simulink model "least_squares_parameter_id"  (R2022a)
settings: Solver=VariableStepAuto  StartTime=0.0  StopTime=10.0  RelTol=1e-3
libraries: simulink x1
settings Model: Creator=mluser  LastModifiedBy=mluser

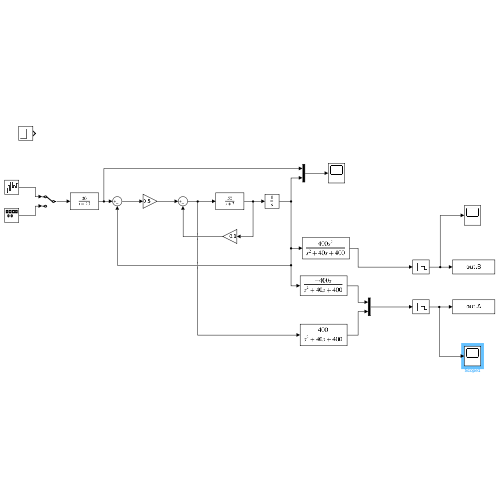
[thumbnail: Simulink's stored preview of the top-level diagram]
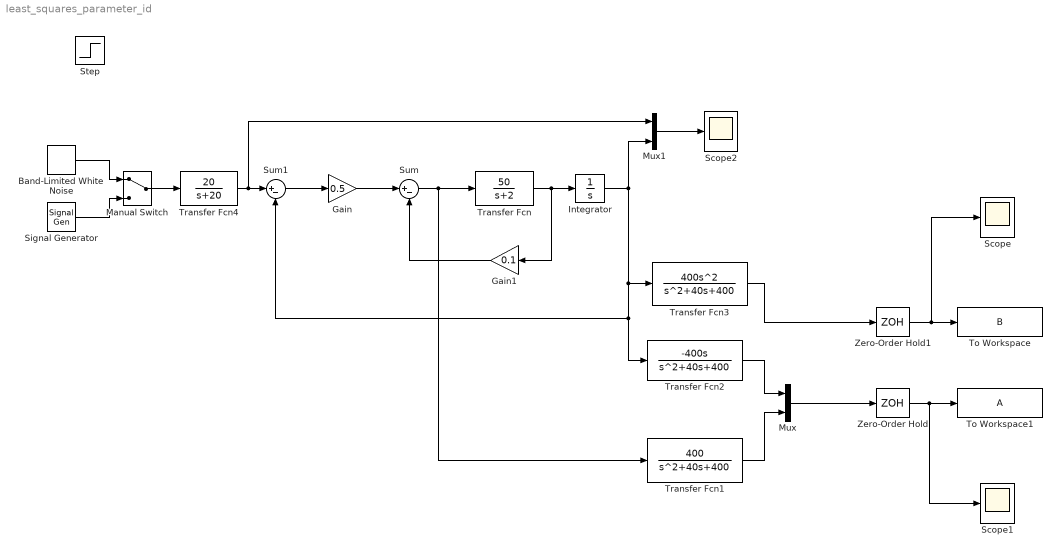
== system least_squares_parameter_id ==
  Band-Limited White Noise : simulink/Sources/Band-Limited White Noise  Cov=[0.1]  Ts=0.1  seed=[23341]
  Gain : Gain  Gain=0.5
  Gain1 : Gain  Gain=0.1
  Integrator : Integrator
  Manual Switch : ManualSwitch
  Mux : Mux  Inputs=2
  Mux1 : Mux  Inputs=2
  Scope : Scope
  Scope1 : Scope
  Scope2 : Scope
  Signal Generator : SignalGenerator  Units=rad/sec
  Step : Step  SampleTime=0
  Sum : Sum  Inputs=|+-
  Sum1 : Sum  Inputs=|+-
  To Workspace : ToWorkspace  VariableName=B  SaveFormat=Timeseries  SampleTime=-1
  To Workspace1 : ToWorkspace  VariableName=A  SaveFormat=Timeseries  SampleTime=-1
  Transfer Fcn : TransferFcn  Numerator=50  Denominator=[1 2]
  Transfer Fcn1 : TransferFcn  Numerator=400  Denominator=[1 40 400]
  Transfer Fcn2 : TransferFcn  Numerator=[-400 0]  Denominator=[1 40 400]
  Transfer Fcn3 : TransferFcn  Numerator=[400 0 0]  Denominator=[1 40 400]
  Transfer Fcn4 : TransferFcn  Numerator=20  Denominator=[1 20]
  Zero-Order Hold : ZeroOrderHold  SampleTime=0.05
  Zero-Order Hold1 : ZeroOrderHold  SampleTime=0.05
  wires:
  Band-Limited White Noise/1 -> Manual Switch/1
  Manual Switch/1 -> Transfer Fcn4/1
  Zero-Order Hold1/1 -> Scope/1, To Workspace/1
  Zero-Order Hold/1 -> Scope1/1, To Workspace1/1
  Mux/1 -> Zero-Order Hold/1
  Mux1/1 -> Scope2/1
  Integrator/1 -> Transfer Fcn3/1, Sum1/2, Transfer Fcn2/1, Mux1/2
  Transfer Fcn/1 -> Gain1/1, Integrator/1
  Sum/1 -> Transfer Fcn1/1, Transfer Fcn/1
  Gain1/1 -> Sum/2
  Sum1/1 -> Gain/1
  Gain/1 -> Sum/1
  Transfer Fcn1/1 -> Mux/2
  Transfer Fcn2/1 -> Mux/1
  Transfer Fcn3/1 -> Zero-Order Hold1/1
  Transfer Fcn4/1 -> Mux1/1, Sum1/1
  Signal Generator/1 -> Manual Switch/2
